simulink model "assignment2"  (Simulink 8.7)
settings: Solver=ode45  StartTime=0.0  StopTime=500  MaxStep=0.01  RelTol=1e-3
values from neighbouring files (symbols this model uses):
  A = [ -0.005131  0        0       0       0 ... (first row only)    [init2.m]
  B = [ -0.629  0.624 ... (first row only)    [init2.m]
  Bd = [ -0.062 -0.067 ... (first row only)    [init2.m]
  C = [ -0.7223 -0.5170  0.3386 -0.1633  0.1121 ... (first row only)    [init2.m]
  g11num = g11num{1,:}    [init2.m]
  g12num = g12num{1,:}    [init2.m]
  g21num = g21num{1,:}    [init2.m]
  g22num = g22num{1,:}    [init2.m]
  k1den = k1den{1,:}    [init2.m]
  k1num = k1num{1,:}    [init2.m]
  k2den = k2den{1,:}    [init2.m]
  k2num = k2num{1,:}    [init2.m]
  Kp1 = 0.5    [init2.m]
  Kp2 = -0.5    [init2.m]
  Ti1 = 2    [init2.m]
  Ti2 = 2    [init2.m]
  Vvar = kv*ones(2,1)    [init2.m]
  Wvar = kw*ones(2,1)    [init2.m]
  y1amp = 1    [init2.m]
  y1freq = 0.005    [init2.m]
  y2amp = 0    [init2.m]
  y2freq = 0.005    [init2.m]
undefined symbols (not defined in the file or in its folder): KFL, lqrK, Wa, Wb, Wc, Wd
settings Model: Creator=anderfo  LastModifiedBy=Sondre
settings DataIOCC: SignalLoggingSaveFormat=ModelDataLogs
settings OptimizationCC: ExpressionDepthLimit=2147483647  InitFltsAndDblsToZero=on
settings DebuggingCC: SaveWithParameterizedLinksMsg=none  SolverPrmCheckMsg=warning  MultiTaskCondExecSysMsg=none  FcnCallInpInsideContextMsg=UseLocalSettings  StateNameClashWarn=warning
settings GRTTargetCC: TargetFcnLib=ansi_tfl_tmw.mat  CombineOutputUpdateFcns=off  GRTInterface=on
settings ConfigComp: CovSFcnEnable=off

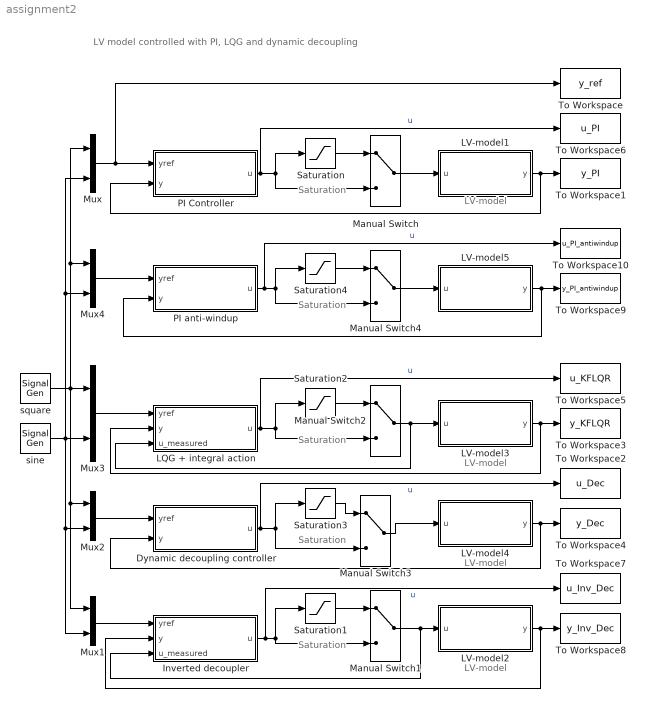
== system assignment2 ==
  note: Saturation
  note: Saturation
  note: Saturation
  note: LV-model
  note: LV-model
  note: LV-model
  note: LV model controlled with PI, LQG and dynamic decoupling
  note: Saturation
  note: LV-model
  note: Saturation
  Dynamic decoupling controller : Subsystem
  Inverted decoupler : Subsystem
  LQG + integral action : Subsystem
  LV-model1 : Subsystem
  LV-model2 : Subsystem
  LV-model3 : Subsystem
  LV-model4 : Subsystem
  LV-model5 : Subsystem
  Manual Switch{,1..4} (5 alike) : ManualSwitch
  Mux{,1..4} (5 alike) : Mux  Inputs=2
  PI Controller : Subsystem
  PI anti-windup : Subsystem
  Saturation{,1..4} (5 alike) : Saturate
  To Workspace : ToWorkspace  VariableName=y_ref  SaveFormat=Structure With Time  SampleTime=-1
  To Workspace1 : ToWorkspace  VariableName=y_PI  SaveFormat=Structure With Time  SampleTime=-1
  To Workspace10 : ToWorkspace  VariableName=u_PI_antiwindup  SaveFormat=Structure With Time  SampleTime=-1
  To Workspace2 : ToWorkspace  VariableName=u_Dec  SaveFormat=Structure With Time  SampleTime=-1
  To Workspace3 : ToWorkspace  VariableName=y_KFLQR  SaveFormat=Structure With Time  SampleTime=-1
  To Workspace4 : ToWorkspace  VariableName=y_Dec  SaveFormat=Structure With Time  SampleTime=-1
  To Workspace5 : ToWorkspace  VariableName=u_KFLQR  SaveFormat=Structure With Time  SampleTime=-1
  To Workspace6 : ToWorkspace  VariableName=u_PI  SaveFormat=Structure With Time  SampleTime=-1
  To Workspace7 : ToWorkspace  VariableName=u_Inv_Dec  SaveFormat=Structure With Time  SampleTime=-1
  To Workspace8 : ToWorkspace  VariableName=y_Inv_Dec  SaveFormat=Structure With Time  SampleTime=-1
  To Workspace9 : ToWorkspace  VariableName=y_PI_antiwindup  SaveFormat=Structure With Time  SampleTime=-1
  sine : SignalGenerator  Amplitude=y2amp  Frequency=y2freq
  square : SignalGenerator  WaveForm=square  Amplitude=y1amp  Frequency=y1freq
  wires:
  Mux/1 -> To Workspace/1, PI Controller/1(yref)
  square/1 -> Mux3/1, Mux2/1, Mux1/1, Mux4/1, Mux/1
  sine/1 -> Mux3/2, Mux2/2, Mux1/2, Mux4/2, Mux/2
  Mux2/1 -> Dynamic decoupling controller/1(yref)
  Mux3/1 -> LQG + integral action/1(yref)
  Manual Switch/1 -> LV-model1/1(u)
  Saturation/1 -> Manual Switch/1
  PI Controller/1(u) -> Manual Switch/2, Saturation/1, To Workspace6/1  "u"
  Manual Switch2/1 -> LQG + integral action/3(u_measured), LV-model3/1(u)
  Saturation2/1 -> Manual Switch2/1
  LQG + integral action/1(u) -> Manual Switch2/2, Saturation2/1, To Workspace5/1  "u"
  Manual Switch3/1 -> LV-model4/1(u)
  Saturation3/1 -> Manual Switch3/1
  Dynamic decoupling controller/1(u) -> Manual Switch3/2, Saturation3/1, To Workspace2/1  "u"
  Mux1/1 -> Inverted decoupler/1(yref)
  LV-model2/1(y) -> To Workspace8/1, Inverted decoupler/2(y)
  Manual Switch1/1 -> LV-model2/1(u), Inverted decoupler/3(u_measured)
  Saturation1/1 -> Manual Switch1/1
  Inverted decoupler/1(u) -> To Workspace7/1, Manual Switch1/2, Saturation1/1  "u"
  LV-model1/1(y) -> To Workspace1/1, PI Controller/2(y)
  LV-model3/1(y) -> To Workspace3/1, LQG + integral action/2(y)
  LV-model4/1(y) -> Dynamic decoupling controller/2(y), To Workspace4/1
  Mux4/1 -> PI anti-windup/1(yref)
  Manual Switch4/1 -> LV-model5/1(u)
  Saturation4/1 -> Manual Switch4/1
  PI anti-windup/1(u) -> To Workspace10/1, Manual Switch4/2, Saturation4/1  "u"
  LV-model5/1(y) -> To Workspace9/1, PI anti-windup/2(y)

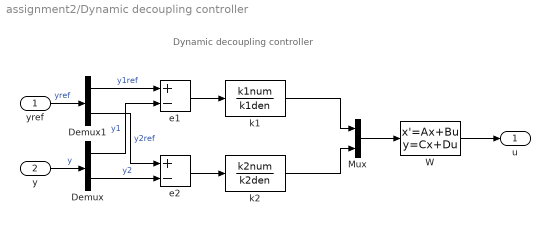
== system assignment2/Dynamic decoupling controller ==
  note: Dynamic decoupling controller
  yref : Inport
  y : Inport  Port=2
  Demux : Demux  Outputs=2
  Demux1 : Demux  Outputs=2
  Mux : Mux  Inputs=2
  W : StateSpace  A=Wa  B=Wb  C=Wc  D=Wd  X0=zeros(1,10)
  e1 : Sum  Inputs=+-
  e2 : Sum  Inputs=+-
  k1 : TransferFcn  Numerator=k1num  Denominator=k1den
  k2 : TransferFcn  Numerator=k2num  Denominator=k2den
  u : Outport
  wires:
  e1/1 -> k1/1
  e2/1 -> k2/1
  y/1 -> Demux/1  "y"
  yref/1 -> Demux1/1  "yref"
  Demux1/1 -> e1/1  "y1ref"
  Demux/1 -> e1/2  "y1"
  Demux1/2 -> e2/1  "y2ref"
  Demux/2 -> e2/2  "y2"
  k1/1 -> Mux/1
  k2/1 -> Mux/2
  Mux/1 -> W/1
  W/1 -> u/1

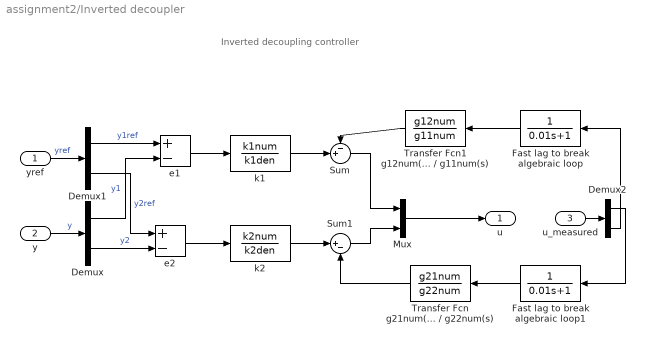
== system assignment2/Inverted decoupler ==
  note: Inverted decoupling controller
  yref : Inport
  y : Inport  Port=2
  u_measured : Inport  Port=3
  Demux : Demux  Outputs=2
  Demux1 : Demux  Outputs=2
  Demux2 : Demux  Outputs=2
  Fast lag to break algebraic loop : TransferFcn  Denominator=[0.01 1]
  Fast lag to break algebraic loop1 : TransferFcn  Denominator=[0.01 1]
  Mux : Mux  Inputs=2
  Sum : Sum  Inputs=-+|
  Sum1 : Sum  Inputs=|+-
  Transfer Fcn g21num(s) / g22num(s) : TransferFcn  Numerator=g21num  Denominator=g22num
  Transfer Fcn1 g12num(s) / g11num(s) : TransferFcn  Numerator=g12num  Denominator=g11num
  e1 : Sum  Inputs=+-
  e2 : Sum  Inputs=+-
  k1 : TransferFcn  Numerator=k1num  Denominator=k1den
  k2 : TransferFcn  Numerator=k2num  Denominator=k2den
  u : Outport
  wires:
  y/1 -> Demux/1  "y"
  yref/1 -> Demux1/1  "yref"
  Demux1/1 -> e1/1  "y1ref"
  Demux/1 -> e1/2  "y1"
  Demux1/2 -> e2/1  "y2ref"
  Demux/2 -> e2/2  "y2"
  Mux/1 -> u/1
  k1/1 -> Sum/2
  k2/1 -> Sum1/1
  Sum1/1 -> Mux/2
  Sum/1 -> Mux/1
  u_measured/1 -> Demux2/1
  Demux2/1 -> Fast lag to break algebraic loop1/1
  Fast lag to break algebraic loop1/1 -> Transfer Fcn g21num(s) / g22num(s)/1
  Transfer Fcn g21num(s) / g22num(s)/1 -> Sum1/2
  Demux2/2 -> Fast lag to break algebraic loop/1
  Fast lag to break algebraic loop/1 -> Transfer Fcn1 g12num(s) / g11num(s)/1
  Transfer Fcn1 g12num(s) / g11num(s)/1 -> Sum/1
  e1/1 -> k1/1
  e2/1 -> k2/1

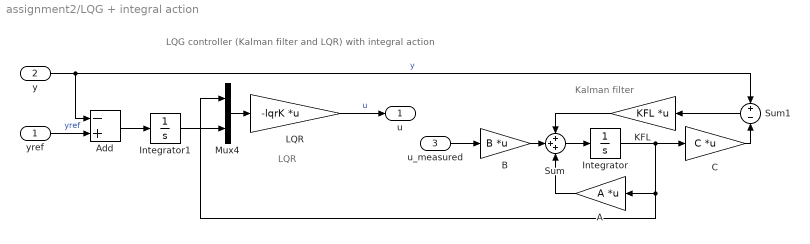
== system assignment2/LQG + integral action ==
  note: LQG controller (Kalman filter and LQR) with integral action
  note: LQR
  note: Kalman filter
  yref : Inport
  y : Inport  Port=2
  u_measured : Inport  Port=3
  A : Gain  Gain=A  Multiplication=Matrix(K*u)
  Add : Sum  Inputs=-+
  B : Gain  Gain=B  Multiplication=Matrix(K*u)
  C : Gain  Gain=C  Multiplication=Matrix(K*u)
  Integrator : Integrator  InitialCondition=[0 0 0 0 0]
  Integrator1 : Integrator  InitialCondition=[0 0]
  KFL : Gain  Gain=KFL  Multiplication=Matrix(K*u)
  LQR : Gain  Gain=-lqrK  Multiplication=Matrix(K*u)
  Mux4 : Mux  Inputs=2
  Sum : Sum  Inputs=+++
  Sum1 : Sum  Inputs=+-
  u : Outport
  wires:
  LQR/1 -> u/1  "u"
  B/1 -> Sum/2
  KFL/1 -> Sum/1
  Sum/1 -> Integrator/1
  A/1 -> Sum/3
  Integrator/1 -> C/1, A/1, Mux4/1
  C/1 -> Sum1/2
  Sum1/1 -> KFL/1
  Mux4/1 -> LQR/1
  u_measured/1 -> B/1
  yref/1 -> Add/2  "yref"
  y/1 -> Sum1/1, Add/1  "y"
  Integrator1/1 -> Mux4/2
  Add/1 -> Integrator1/1

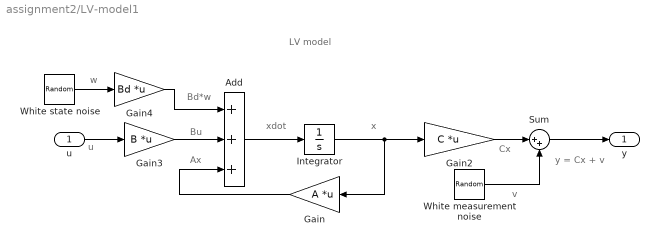
== system assignment2/LV-model1 ==
  note: v
  note: w
  note: y = Cx + v
  note: Ax
  note: u
  note: x
  note: xdot
  note: Bd*w
  note: Bu
  note: Cx
  note: LV model
  u : Inport
  Add : Sum  Inputs=+++
  Gain : Gain  Gain=A  Multiplication=Matrix(K*u)
  Gain2 : Gain  Gain=C  Multiplication=Matrix(K*u)
  Gain3 : Gain  Gain=B  Multiplication=Matrix(K*u)
  Gain4 : Gain  Gain=Bd  Multiplication=Matrix(K*u)
  Integrator : Integrator
  Sum : Sum  Inputs=|++
  White measurement noise : RandomNumber  Variance=Vvar  Seed=[3 4]  SampleTime=0
  White state noise : RandomNumber  Variance=Wvar  Seed=[1 2]  SampleTime=0
  y : Outport
  wires:
  u/1 -> Gain3/1
  White measurement noise/1 -> Sum/2
  Sum/1 -> y/1
  Gain2/1 -> Sum/1
  White state noise/1 -> Gain4/1
  Add/1 -> Integrator/1
  Gain/1 -> Add/3
  Gain3/1 -> Add/2
  Integrator/1 -> Gain2/1, Gain/1
  Gain4/1 -> Add/1

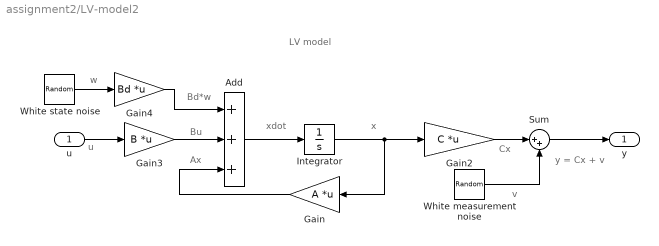
== system assignment2/LV-model2 ==
  note: v
  note: w
  note: y = Cx + v
  note: Ax
  note: u
  note: x
  note: xdot
  note: Bd*w
  note: Bu
  note: Cx
  note: LV model
  u : Inport
  Add : Sum  Inputs=+++
  Gain : Gain  Gain=A  Multiplication=Matrix(K*u)
  Gain2 : Gain  Gain=C  Multiplication=Matrix(K*u)
  Gain3 : Gain  Gain=B  Multiplication=Matrix(K*u)
  Gain4 : Gain  Gain=Bd  Multiplication=Matrix(K*u)
  Integrator : Integrator
  Sum : Sum  Inputs=|++
  White measurement noise : RandomNumber  Variance=Vvar  Seed=[3 4]  SampleTime=0
  White state noise : RandomNumber  Variance=Wvar  Seed=[1 2]  SampleTime=0
  y : Outport
  wires:
  u/1 -> Gain3/1
  White measurement noise/1 -> Sum/2
  Sum/1 -> y/1
  Gain2/1 -> Sum/1
  White state noise/1 -> Gain4/1
  Add/1 -> Integrator/1
  Gain/1 -> Add/3
  Gain3/1 -> Add/2
  Integrator/1 -> Gain2/1, Gain/1
  Gain4/1 -> Add/1

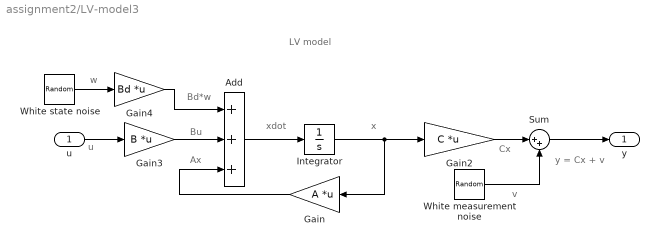
== system assignment2/LV-model3 ==
  note: v
  note: w
  note: y = Cx + v
  note: Ax
  note: u
  note: x
  note: xdot
  note: Bd*w
  note: Bu
  note: Cx
  note: LV model
  u : Inport
  Add : Sum  Inputs=+++
  Gain : Gain  Gain=A  Multiplication=Matrix(K*u)
  Gain2 : Gain  Gain=C  Multiplication=Matrix(K*u)
  Gain3 : Gain  Gain=B  Multiplication=Matrix(K*u)
  Gain4 : Gain  Gain=Bd  Multiplication=Matrix(K*u)
  Integrator : Integrator
  Sum : Sum  Inputs=|++
  White measurement noise : RandomNumber  Variance=Vvar  Seed=[3 4]  SampleTime=0
  White state noise : RandomNumber  Variance=Wvar  Seed=[1 2]  SampleTime=0
  y : Outport
  wires:
  u/1 -> Gain3/1
  White measurement noise/1 -> Sum/2
  Sum/1 -> y/1
  Gain2/1 -> Sum/1
  White state noise/1 -> Gain4/1
  Add/1 -> Integrator/1
  Gain/1 -> Add/3
  Gain3/1 -> Add/2
  Integrator/1 -> Gain2/1, Gain/1
  Gain4/1 -> Add/1

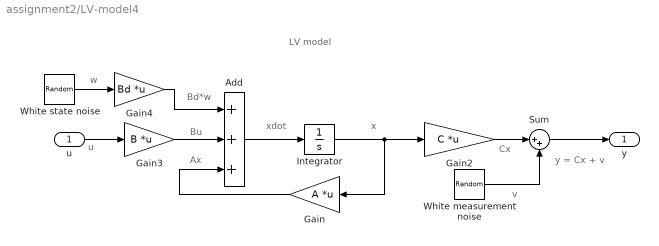
== system assignment2/LV-model4 ==
  note: v
  note: w
  note: y = Cx + v
  note: Ax
  note: u
  note: x
  note: xdot
  note: Bd*w
  note: Bu
  note: Cx
  note: LV model
  u : Inport
  Add : Sum  Inputs=+++
  Gain : Gain  Gain=A  Multiplication=Matrix(K*u)
  Gain2 : Gain  Gain=C  Multiplication=Matrix(K*u)
  Gain3 : Gain  Gain=B  Multiplication=Matrix(K*u)
  Gain4 : Gain  Gain=Bd  Multiplication=Matrix(K*u)
  Integrator : Integrator
  Sum : Sum  Inputs=|++
  White measurement noise : RandomNumber  Variance=Vvar  Seed=[3 4]  SampleTime=0
  White state noise : RandomNumber  Variance=Wvar  Seed=[1 2]  SampleTime=0
  y : Outport
  wires:
  u/1 -> Gain3/1
  White measurement noise/1 -> Sum/2
  Sum/1 -> y/1
  Gain2/1 -> Sum/1
  White state noise/1 -> Gain4/1
  Add/1 -> Integrator/1
  Gain/1 -> Add/3
  Gain3/1 -> Add/2
  Integrator/1 -> Gain2/1, Gain/1
  Gain4/1 -> Add/1

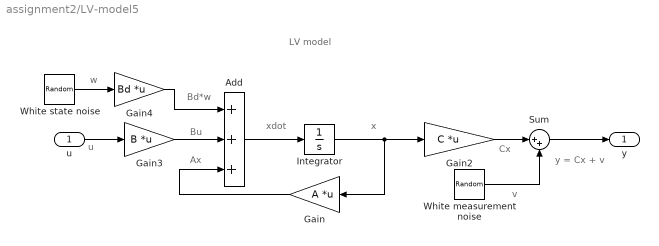
== system assignment2/LV-model5 ==
  note: v
  note: w
  note: y = Cx + v
  note: Ax
  note: u
  note: x
  note: xdot
  note: Bd*w
  note: Bu
  note: Cx
  note: LV model
  u : Inport
  Add : Sum  Inputs=+++
  Gain : Gain  Gain=A  Multiplication=Matrix(K*u)
  Gain2 : Gain  Gain=C  Multiplication=Matrix(K*u)
  Gain3 : Gain  Gain=B  Multiplication=Matrix(K*u)
  Gain4 : Gain  Gain=Bd  Multiplication=Matrix(K*u)
  Integrator : Integrator
  Sum : Sum  Inputs=|++
  White measurement noise : RandomNumber  Variance=Vvar  Seed=[3 4]  SampleTime=0
  White state noise : RandomNumber  Variance=Wvar  Seed=[1 2]  SampleTime=0
  y : Outport
  wires:
  u/1 -> Gain3/1
  White measurement noise/1 -> Sum/2
  Sum/1 -> y/1
  Gain2/1 -> Sum/1
  White state noise/1 -> Gain4/1
  Add/1 -> Integrator/1
  Gain/1 -> Add/3
  Gain3/1 -> Add/2
  Integrator/1 -> Gain2/1, Gain/1
  Gain4/1 -> Add/1

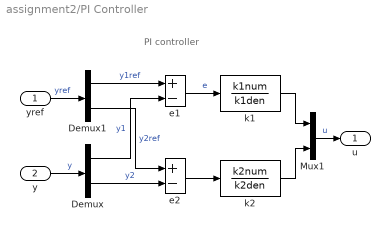
== system assignment2/PI Controller ==
  note: PI controller
  yref : Inport
  y : Inport  Port=2
  Demux : Demux  Outputs=2
  Demux1 : Demux  Outputs=2
  Mux1 : Mux  Inputs=2
  e1 : Sum  Inputs=+-
  e2 : Sum  Inputs=+-
  k1 : TransferFcn  Numerator=k1num  Denominator=k1den
  k2 : TransferFcn  Numerator=k2num  Denominator=k2den
  u : Outport
  wires:
  e1/1 -> k1/1  "e"
  k1/1 -> Mux1/1
  k2/1 -> Mux1/2
  Mux1/1 -> u/1  "u"
  y/1 -> Demux/1  "y"
  yref/1 -> Demux1/1  "yref"
  Demux1/1 -> e1/1  "y1ref"
  Demux/1 -> e1/2  "y1"
  Demux1/2 -> e2/1  "y2ref"
  Demux/2 -> e2/2  "y2"
  e2/1 -> k2/1

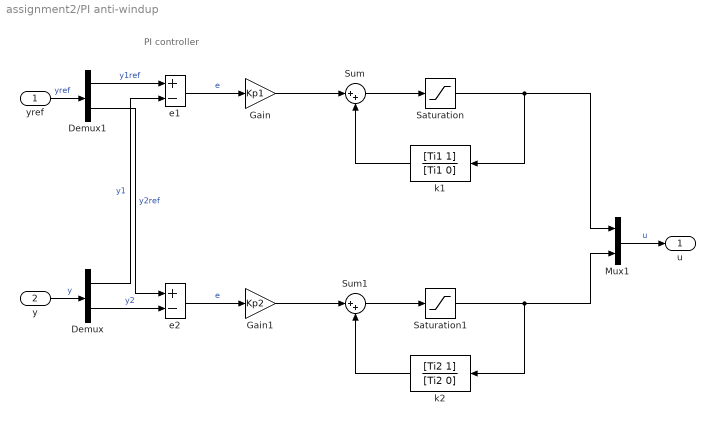
== system assignment2/PI anti-windup ==
  note: PI controller
  yref : Inport
  y : Inport  Port=2
  Demux : Demux  Outputs=2
  Demux1 : Demux  Outputs=2
  Gain : Gain  Gain=Kp1
  Gain1 : Gain  Gain=Kp2
  Mux1 : Mux  Inputs=2
  Saturation : Saturate
  Saturation1 : Saturate
  Sum : Sum  Inputs=|++
  Sum1 : Sum  Inputs=|++
  e1 : Sum  Inputs=+-
  e2 : Sum  Inputs=+-
  k1 : TransferFcn  Numerator=[Ti1 1]  Denominator=[Ti1 0]
  k2 : TransferFcn  Numerator=[Ti2 1]  Denominator=[Ti2 0]
  u : Outport
  wires:
  Mux1/1 -> u/1  "u"
  y/1 -> Demux/1  "y"
  yref/1 -> Demux1/1  "yref"
  Demux1/1 -> e1/1  "y1ref"
  Demux/1 -> e1/2  "y1"
  Demux1/2 -> e2/1  "y2ref"
  Demux/2 -> e2/2  "y2"
  e1/1 -> Gain/1  "e"
  Sum/1 -> Saturation/1
  Gain/1 -> Sum/1
  k1/1 -> Sum/2
  Saturation/1 -> k1/1, Mux1/1
  e2/1 -> Gain1/1  "e"
  Sum1/1 -> Saturation1/1
  Gain1/1 -> Sum1/1
  k2/1 -> Sum1/2
  Saturation1/1 -> k2/1, Mux1/2
